simulink model "reg_lqr2_2014"  (Simulink 8.3)
settings: Solver=ode4  StartTime=0.0  StopTime=30  FixedStep=0.001  RelTol=1e-3
values from neighbouring files (symbols this model uses):
  A = [0 1 ... (first row only)    [cel.m]    (also in celPID.m; min_PID.m; pod_discPID.m; por_model_obiekt_osX.m)
  Al = [0  1     0 0 ... (first row only)    [cel.m]    (also in req_lqr.m; zobserwatorem.m)
  B = [0; k/omega0^2]    [cel.m]    (also in celPID.m; min_PID.m; pod_discPID.m; por_model_obiekt_osX.m)
  Bl = [0; Km/T; 0; K*Km*omega^2/T]    [cel.m]    (also in req_lqr.m; zobserwatorem.m)
  C = [1 0]    [cel.m]    (also in celPID.m; min_PID.m; pod_discPID.m; por_model_obiekt_osX.m)
  Cl = [1 0 0 0 ... (first row only)    [cel.m]    (also in req_lqr.m; zobserwatorem.m)
  D = 0    [cel.m]    (also in celPID.m; min_PID.m; pod_discPID.m; por_model_obiekt_osX.m)
  Klqr = lqr(Al,Bl,Q,R)    [cel.m]    (also in req_lqr.m)
  L = transpose(place(transpose(Al),transpose(Cl), [-11 -10 -9 -11]))    [cel.m]    (also in req_lqr.m; zobserwatorem.m)
  limitT = 0.05    [cel.m]    (also in celPID.m; dane.m; pod_discPID.m)
  X0 = [0 0 0 0]    [cel.m]    (also in celPID.m = [0 0]; min_PID.m = [0 0]; pod_discPID.m = [0 0]; por_model_obiekt_osX.m = [0 0])
settings Model: Creator=Maciek  LastModifiedBy=Maciek  CovModelRefEnable=off  CovSFcnEnable=on
settings DataIOCC: LimitDataPoints=off  SaveFormat=StructureWithTime  SignalLoggingSaveFormat=Dataset
settings DebuggingCC: UnderspecifiedInitializationDetection=Simplified  MergeDetectMultiDrivingBlocksExec=error  SolverPrmCheckMsg=none  FrameProcessingCompatibilityMsg=error  StateNameClashWarn=none
settings HardwareCC: ProdBitPerPointer=64  ProdLargestAtomicFloat=Float  ProdIntDivRoundTo=Zero  ProdEndianess=LittleEndian  ProdHWDeviceType=Specified
settings ModelReferenceCC: PropagateSignalLabelsOutOfModel=on
settings GRTTargetCC: CombineOutputUpdateFcns=on  GRTInterface=off

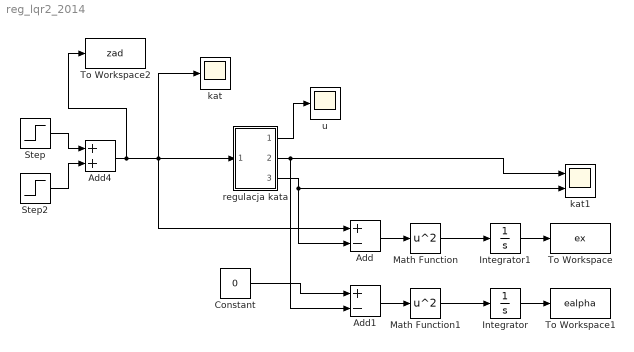
== system reg_lqr2_2014 ==
  Add : Sum  Inputs=+-
  Add1 : Sum  Inputs=+-
  Add4 : Sum
  Constant : Constant  Value=0
  Integrator : Integrator
  Integrator1 : Integrator
  Math Function : Math  Operator=square  SaturateOnIntegerOverflow=on
  Math Function1 : Math  Operator=square  SaturateOnIntegerOverflow=on
  Step : Step  After=0.2  SampleTime=0
  Step2 : Step  Time=40  After=-0.7  SampleTime=0
  To Workspace : ToWorkspace  VariableName=ex  SampleTime=-1
      settings: MaxDataPoints=1
  To Workspace1 : ToWorkspace  VariableName=ealpha  SampleTime=-1
      settings: MaxDataPoints=1
  To Workspace2 : ToWorkspace  VariableName=zad  SaveFormat=Timeseries  SampleTime=-1
  kat : Scope
      settings: TimeRange=auto  MaxDataPoints=5000  SaveName=kat  YMin=-0.26466  YMax=0.30003  SampleTime=-1
  kat1 : Scope  NumInputPorts=2
      settings: TimeRange=auto  MaxDataPoints=5000  SaveName=obs_y  YMin=-0.04169~-0.0249  YMax=0.06739~0.22414  SampleTime=-1
  regulacja kata : Subsystem
  u : Scope
      settings: TimeRange=auto  MaxDataPoints=5000  SaveName=ScopeData4  YMin=-165.90034  YMax=614.77228  SampleTime=-1
  wires:
  Step/1 -> Add4/1
  Step2/1 -> Add4/2
  regulacja kata/1(Out1) -> u/1
  regulacja kata/2(alpha) -> Add1/2, kat1/1
  regulacja kata/3(pol) -> Add/2, kat1/2
  Add4/1 -> To Workspace2/1, kat/1, Add/1, regulacja kata/1(zad)
  Add/1 -> Math Function/1
  Add1/1 -> Math Function1/1
  Math Function1/1 -> Integrator/1
  Math Function/1 -> Integrator1/1
  Integrator1/1 -> To Workspace/1
  Integrator/1 -> To Workspace1/1
  Constant/1 -> Add1/1

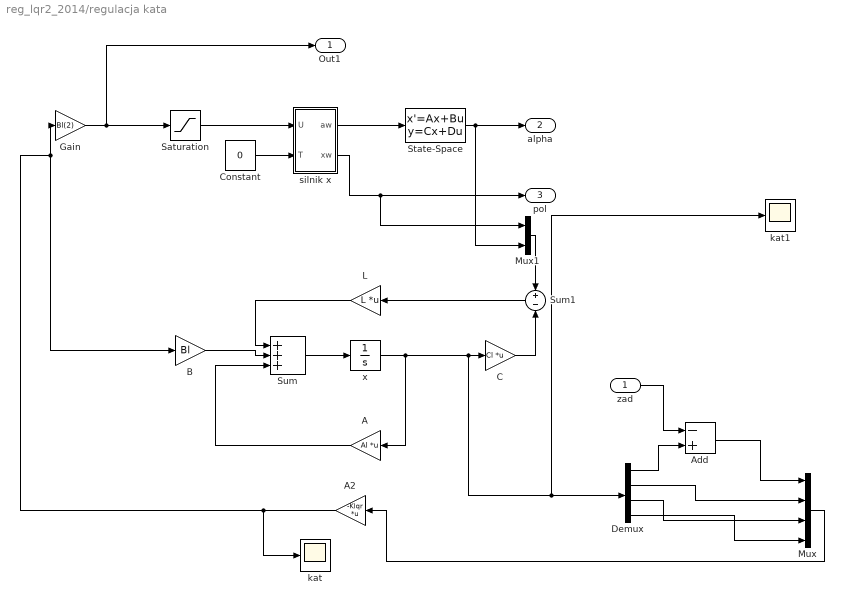
== system reg_lqr2_2014/regulacja kata ==
  zad : Inport
  A : Gain  Gain=Al  Multiplication=Matrix(K*u) (u vector)
  A2 : Gain  Gain=-Klqr  Multiplication=Matrix(K*u) (u vector)
  Add : Sum  Inputs=-+
  B : Gain  Gain=Bl
  C : Gain  Gain=Cl  Multiplication=Matrix(K*u) (u vector)
  Constant : Constant  Value=0
  Demux : Demux
  Gain : Gain  Gain=Bl(2)
  L : Gain  Gain=L  Multiplication=Matrix(K*u) (u vector)
  Mux : Mux
  Mux1 : Mux  Inputs=2
  Saturation : Saturate  UpperLimit=1  LowerLimit=-1
  State-Space : StateSpace  A=A  B=B  C=C  D=D  X0=[ 0 0]
  Sum : Sum  Inputs=+++
  Sum1 : Sum  Inputs=+-
  kat : Scope
      settings: TimeRange=auto  MaxDataPoints=5000  SaveName=kat1  YMin=-0.00119  YMax=0.0106  SampleTime=-1
  kat1 : Scope
      settings: TimeRange=auto  MaxDataPoints=5000  SaveName=kat2  YMin=-0.43926  YMax=0.46338  SampleTime=-1
  silnik x : Subsystem
  x : Integrator  InitialCondition=X0
  Out1 : Outport
  alpha : Outport  Port=2
  pol : Outport  Port=3
  wires:
  silnik x/1(aw) -> State-Space/1
  silnik x/2(xw) -> Mux1/1, pol/1
  zad/1 -> Add/1
  Saturation/1 -> silnik x/1(U)
  Constant/1 -> silnik x/2(T)
  State-Space/1 -> Mux1/2, alpha/1
  Sum/1 -> x/1
  x/1 -> A/1, kat1/1, Demux/1, C/1
  A/1 -> Sum/3
  C/1 -> Sum1/2
  Sum1/1 -> L/1
  L/1 -> Sum/1
  B/1 -> Sum/2
  A2/1 -> kat/1, Gain/1, B/1
  Mux1/1 -> Sum1/1
  Gain/1 -> Out1/1, Saturation/1
  Demux/1 -> Add/2
  Add/1 -> Mux/1
  Demux/2 -> Mux/2
  Demux/3 -> Mux/3
  Demux/4 -> Mux/4
  Mux/1 -> A2/1

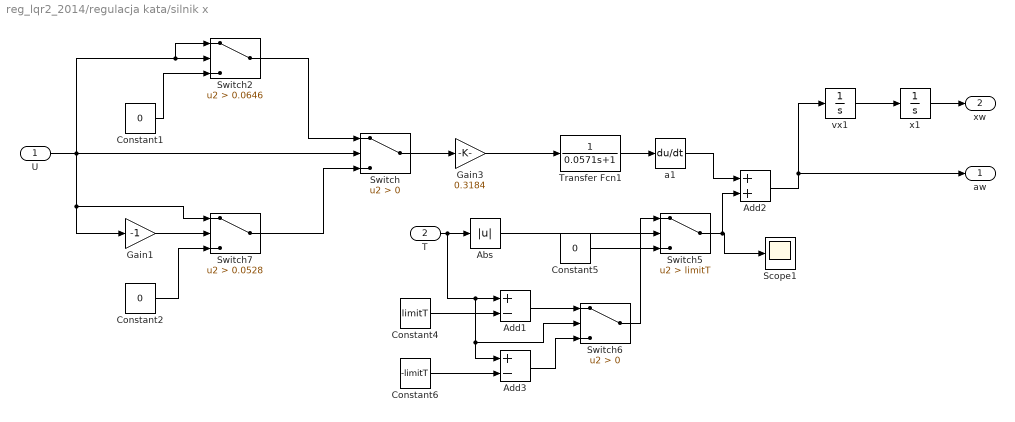
== system reg_lqr2_2014/regulacja kata/silnik x ==
  U : Inport
  T : Inport  Port=2
  Abs : Abs
  Add1 : Sum  Inputs=+-
  Add2 : Sum
  Add3 : Sum  Inputs=+-
  Constant1 : Constant  Value=0
  Constant2 : Constant  Value=0
  Constant4 : Constant  Value=limitT
  Constant5 : Constant  Value=0
  Constant6 : Constant  Value=-limitT
  Gain1 : Gain  Gain=-1
  Gain3 : Gain  Gain=0.3184
  Scope1 : Scope
      settings: TimeRange=auto  MaxDataPoints=5000  SaveToWorkspace=off  SaveName=ScopeData2  YMin=-0.45032  YMax=0.28533  SampleTime=-1
  Switch : Switch  Criteria=u2 > Threshold
  Switch2 : Switch  Criteria=u2 > Threshold  Threshold=0.0646
  Switch5 : Switch  Criteria=u2 > Threshold  Threshold=limitT
  Switch6 : Switch  Criteria=u2 > Threshold
  Switch7 : Switch  Criteria=u2 > Threshold  Threshold=0.0528
  Transfer Fcn1 : TransferFcn  Numerator=1  Denominator=[0.0571 1]
  a1 : Derivative
  vx1 : Integrator
  x1 : Integrator
  aw : Outport
  xw : Outport  Port=2
  wires:
  Constant1/1 -> Switch2/3
  Switch2/1 -> Switch/1
  Constant2/1 -> Switch7/3
  U/1 -> Switch7/1, Gain1/1, Switch2/1, Switch2/2, Switch/2
  Switch7/1 -> Switch/3
  Gain1/1 -> Switch7/2
  Transfer Fcn1/1 -> a1/1
  x1/1 -> xw/1
  vx1/1 -> x1/1
  Gain3/1 -> Transfer Fcn1/1
  Add2/1 -> aw/1, vx1/1
  a1/1 -> Add2/1
  Switch5/1 -> Add2/2, Scope1/1
  T/1 -> Add3/1, Switch6/2, Add1/1, Abs/1
  Abs/1 -> Switch5/2
  Constant4/1 -> Add1/2
  Constant5/1 -> Switch5/3
  Switch6/1 -> Switch5/1
  Add1/1 -> Switch6/1
  Constant6/1 -> Add3/2
  Add3/1 -> Switch6/3
  Switch/1 -> Gain3/1
